simulink model "Demo919"  (R2018b)
settings: Solver=ode3  StartTime=0.0  StopTime=10  FixedStep=0.0005  RelTol=1e-3  EnableMultiTasking=on
values from neighbouring files (symbols this model uses):
  ADS1 = [1000 4000]    [data_new1.m]
  ADS2 = [900 4100]    [data_new1.m]
  br_opening = [0 20 40 60 80 100]    [data_new1.m]
  BRAKE = [485 1288 2091 2894 3697 4500]    [data_new1.m]
  InerWheel_Angle = [0 0.001 0.502 1.006 1.514 2.024 2.538 3.055 3.575 4.098 4.625 5.155 5.689 6.226 6.767 7.311 7.859 8.411 8.967 9.527 10.091 10.659 11.231 11.807 12.387 12.972 13.561 14.154 14.752 15.354 15.961 16.572 17.187 17.807 18.432 19.062 19.696 20.334 20.977 21.625 22.277 22.934 23.596 24.262 24.932 25.607 26.286 26.970 27.657 28.349 29.045 29.745 30.448 31.155 31.866]    [data_new1.m]
  OuterWheel_Angle = [0 0.001 0.501 1.001 1.501 2.001 2.501	3.001 3.501	4.001 4.501	5.001 5.501	6.001 6.501	7.001 7.501	8.001 8.501	9.001 9.501	10.001 10.501 11.001 11.501 12.001 12.501 13.001 13.501	14.001 14.501 15.001 15.501 16.001 16.501 17.001 17.501 18.001 18.501 19.001 19.501	20.001 20.501 21.001 21.501	22.001 22.501 23.001 23.501	24.001 24.501 25.001 25.501 26.001 26.501]    [data_new1.m]
  PUMP = [0 1000 2000 3000 4000 5000]    [data_new1.m]
  SteeringAngle_Cal = [-90 0 90]    [data_new1.m]
  SteeringAngle_Sensor = [640 1840 3041]    [data_new1.m]
  th_opening = [0 100]    [data_new1.m]
undefined symbols (not defined in the file or in its folder): D, I_AN06_5V, I_AN08_5V, I_AN09_5V, I_AN10_5V, I_HALL1, I_HALL2, I_SW01_L, I_SW10_L, I_SW11_H, I_SW12_H, I_SW13_H, I_SW14_H, I_SW15_H, I_SW16_H, I_SW17_H, I_SW18_H, I_SW19_H, I_SW20_H, O_PWM1_LS0A7, O_PWM2_LS0A7, O_SW02_LS0A4, O_SW13_HS1A, O_SW14_HS1A
libraries: ec5744lib x137, simulink x20, canmsglib x11
(part 4 of 5)

== system Demo919/Function-Call Subsystem1/Torque_Control/kongzhimokuai/FZ ==
  In1 : Inport
  In2 : Inport  Port=2
  Add3 : Sum
  Add4 : Sum
  Add7 : Sum
  Add8 : Sum  Inputs=+-
  Constant : Constant  Value=930
  Constant2 : Constant  Value=930
  Gain1 : Gain
  Gain11 : Gain
  Gain5 : Gain  Gain=33.17
  Gain6 : Gain  Gain=190.19
  Gain8 : Gain  Gain=33.17
  Gain9 : Gain  Gain=190.19
  k : Gain  Gain=14
  k1 : Gain  Gain=14
  Out1 : Outport
  Out2 : Outport  Port=2
  wires:
  Constant/1 -> Add7/2
  Add7/1 -> Add8/1
  k/1 -> Gain5/1
  Gain5/1 -> Add7/1
  Gain6/1 -> Add8/2
  Gain11/1 -> Gain6/1
  Add8/1 -> Out1/1
  In1/1 -> k1/1, k/1
  Gain1/1 -> Gain9/1
  Gain9/1 -> Add4/2
  Gain8/1 -> Add3/1
  k1/1 -> Gain8/1
  In2/1 -> Gain1/1, Gain11/1
  Add3/1 -> Add4/1
  Constant2/1 -> Add3/2
  Add4/1 -> Out2/1

== system Demo919/Function-Call Subsystem1/Torque_Control/kongzhimokuai/Filter1 ==
  note: 均值滤波器
  In1 : Inport
  Add2 : Sum  Inputs=-+-
  Gain2 : Gain  Gain=1/4
  MinMax : MinMax
  MinMax1 : MinMax  Function=max
  Sum of Elements : Sum  Inputs=+
  Tapped Delay : simulink/Discrete/Tapped Delay  vinit=0  samptime=-1  NumDelays=4  DelayOrder=Oldest  includeCurrent=off
  Out1 : Outport
  wires:
  Tapped Delay/1 -> Sum of Elements/1, MinMax1/1, MinMax/1
  Sum of Elements/1 -> Add2/2
  Gain2/1 -> Out1/1
  MinMax1/1 -> Add2/1
  MinMax/1 -> Add2/3
  Add2/1 -> Gain2/1
  In1/1 -> Tapped Delay/1

== system Demo919/Function-Call Subsystem1/Torque_Control/kongzhimokuai/Filter2 ==
  note: 均值滤波器
  In1 : Inport
  Add2 : Sum  Inputs=-+-
  Gain2 : Gain  Gain=1/4
  MinMax : MinMax
  MinMax1 : MinMax  Function=max
  Sum of Elements : Sum  Inputs=+
  Tapped Delay : simulink/Discrete/Tapped Delay  vinit=0.0  samptime=-1  NumDelays=6  DelayOrder=Oldest  includeCurrent=off
  Out1 : Outport
  wires:
  In1/1 -> Tapped Delay/1
  Add2/1 -> Gain2/1
  MinMax/1 -> Add2/3
  MinMax1/1 -> Add2/1
  Gain2/1 -> Out1/1
  Sum of Elements/1 -> Add2/2
  Tapped Delay/1 -> MinMax/1, MinMax1/1, Sum of Elements/1

== system Demo919/Function-Call Subsystem1/Torque_Control/kongzhimokuai/Filter3 ==
  note: 均值滤波器
  In1 : Inport
  Add2 : Sum  Inputs=-+-
  Gain2 : Gain  Gain=1/4
  MinMax : MinMax
  MinMax1 : MinMax  Function=max
  Sum of Elements : Sum  Inputs=+
  Tapped Delay : simulink/Discrete/Tapped Delay  vinit=0.0  samptime=-1  NumDelays=6  DelayOrder=Oldest  includeCurrent=off
  Out1 : Outport
  wires:
  Tapped Delay/1 -> Sum of Elements/1, MinMax1/1, MinMax/1
  Sum of Elements/1 -> Add2/2
  Gain2/1 -> Out1/1
  MinMax1/1 -> Add2/1
  MinMax/1 -> Add2/3
  Add2/1 -> Gain2/1
  In1/1 -> Tapped Delay/1

== system Demo919/Function-Call Subsystem1/Torque_Control/kongzhimokuai/Filter4 ==
  note: 均值滤波器
  In1 : Inport
  Add2 : Sum  Inputs=-+-
  Gain2 : Gain  Gain=1/4  OutDataTypeStr=double
  MinMax : MinMax
  MinMax1 : MinMax  Function=max
  Sum of Elements : Sum  Inputs=+
  Tapped Delay : simulink/Discrete/Tapped Delay  vinit=0  samptime=-1  NumDelays=4  DelayOrder=Oldest  includeCurrent=off
  Out1 : Outport
  wires:
  In1/1 -> Tapped Delay/1
  Add2/1 -> Gain2/1
  MinMax/1 -> Add2/3
  MinMax1/1 -> Add2/1
  Gain2/1 -> Out1/1
  Sum of Elements/1 -> Add2/2
  Tapped Delay/1 -> MinMax/1, MinMax1/1, Sum of Elements/1

== system Demo919/Function-Call Subsystem1/Torque_Control/kongzhimokuai/Filter5 ==
  note: 均值滤波器
  In1 : Inport
  Add2 : Sum  Inputs=-+-
  MinMax : MinMax
  MinMax1 : MinMax  Function=max
  Sum of Elements : Sum  Inputs=+
  Tapped Delay : simulink/Discrete/Tapped Delay  vinit=0  samptime=-1  NumDelays=3  DelayOrder=Oldest  includeCurrent=off
  Out1 : Outport
  wires:
  Tapped Delay/1 -> Sum of Elements/1, MinMax1/1, MinMax/1
  Sum of Elements/1 -> Add2/2
  Add2/1 -> Out1/1
  MinMax1/1 -> Add2/1
  MinMax/1 -> Add2/3
  In1/1 -> Tapped Delay/1

== system Demo919/Function-Call Subsystem1/Torque_Control/kongzhimokuai/Filter6 ==
  note: 均值滤波器
  In1 : Inport
  Add2 : Sum  Inputs=-+-
  MinMax : MinMax
  MinMax1 : MinMax  Function=max
  Sum of Elements : Sum  Inputs=+
  Tapped Delay : simulink/Discrete/Tapped Delay  vinit=0  samptime=-1  NumDelays=3  DelayOrder=Oldest  includeCurrent=off
  Out1 : Outport
  wires:
  Tapped Delay/1 -> Sum of Elements/1, MinMax1/1, MinMax/1
  Sum of Elements/1 -> Add2/2
  Add2/1 -> Out1/1
  MinMax1/1 -> Add2/1
  MinMax/1 -> Add2/3
  In1/1 -> Tapped Delay/1

== system Demo919/Function-Call Subsystem1/Torque_Control/kongzhimokuai/Fx ==
  In1 : Inport
  In2 : Inport  Port=2
  Add7 : Sum  Inputs=-+
  Add8 : Sum  Inputs=+-
  From96 : From  Commented=on  GotoTag=RolA21
  From97 : From  Commented=on  GotoTag=RolA22
  Gain5 : Gain  Gain=3.9
  Gain6 : Gain  Gain=3.9
  Jw : Constant  Commented=on  Value=0.235
  Jw1 : Constant  Commented=on  Value=0.235
  Product10 : Product  Commented=on
  Product11 : Product  Commented=on
  Out1 : Outport
  Out2 : Outport  Port=2
  wires:
  From96/1 -> Product10/2
  Gain5/1 -> Add8/1
  Product11/1 -> Add8/2
  Gain6/1 -> Add7/2
  Jw/1 -> Product10/1
  Jw1/1 -> Product11/2
  Product10/1 -> Add7/1
  From97/1 -> Product11/1
  In2/1 -> Gain5/1
  In1/1 -> Gain6/1
  Add7/1 -> Out1/1
  Add8/1 -> Out2/1

== system Demo919/Function-Call Subsystem1/Torque_Control/kongzhimokuai/Kalman_Filer ==
  In1 : Inport
  Data Type Conversion : DataTypeConversion  OutDataTypeStr=single
  Data Type Conversion1 : DataTypeConversion  OutDataTypeStr=single
  Delay : Delay  DelayLength=1  InitialCondition=0
  Delay1 : Delay  DelayLength=1  InitialCondition=0
  MATLAB Function : MATLAB Function  TreatAsAtomicUnit=on
  Out1 : Outport
  wires:
  In1/1 -> Data Type Conversion/1
  Data Type Conversion1/1 -> MATLAB Function/2(prevData)
  Data Type Conversion/1 -> MATLAB Function/1(inData)
  Delay/1 -> Data Type Conversion1/1
  MATLAB Function/1(inData_Output) -> Out1/1, Delay/1
  Delay1/1 -> MATLAB Function/3(Error)
  MATLAB Function/2(Error_Last) -> Delay1/1

== system Demo919/Function-Call Subsystem1/Torque_Control/kongzhimokuai/Kalman_Filer1 ==
  In1 : Inport
  Data Type Conversion : DataTypeConversion  OutDataTypeStr=single
  Data Type Conversion1 : DataTypeConversion  OutDataTypeStr=single
  Delay : Delay  DelayLength=1  InitialCondition=0
  Delay1 : Delay  DelayLength=1  InitialCondition=0
  MATLAB Function : MATLAB Function  TreatAsAtomicUnit=on
  Out1 : Outport
  wires:
  MATLAB Function/2(Error_Last) -> Delay1/1
  Delay1/1 -> MATLAB Function/3(Error)
  MATLAB Function/1(inData_Output) -> Delay/1, Out1/1
  Delay/1 -> Data Type Conversion1/1
  Data Type Conversion/1 -> MATLAB Function/1(inData)
  Data Type Conversion1/1 -> MATLAB Function/2(prevData)
  In1/1 -> Data Type Conversion/1

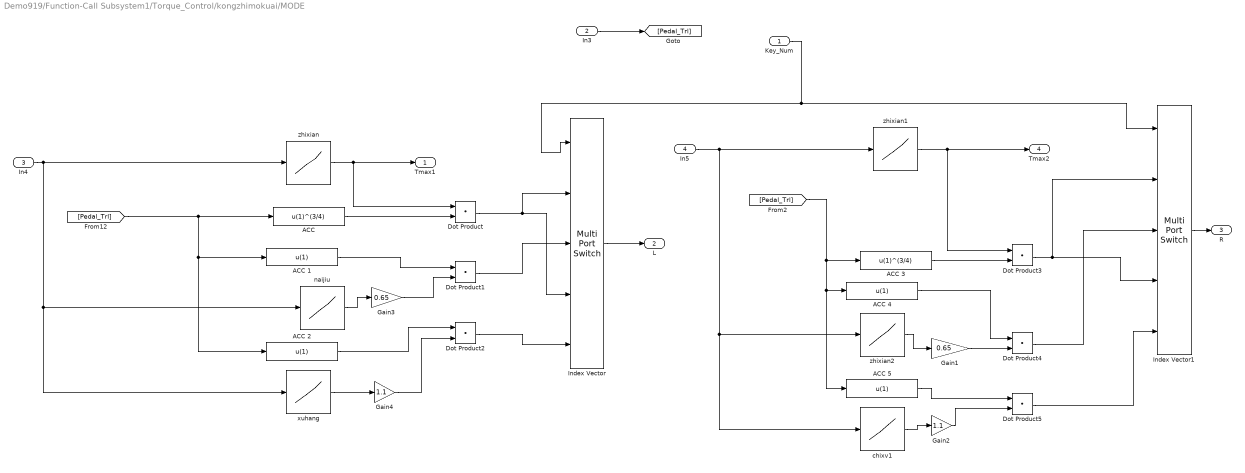
== system Demo919/Function-Call Subsystem1/Torque_Control/kongzhimokuai/MODE ==
  Key_Num : Inport
  In3 : Inport  Port=2
  In4 : Inport  Port=3
  In5 : Inport  Port=4
  "ACC " : Fcn  Expr=u(1)^(3/4)
  ACC {1..2,4..5} (4 alike) : Fcn  Expr=u(1)
  ACC 3 : Fcn  Expr=u(1)^(3/4)
  Dot Product{,1..5} (6 alike) : DotProduct  InputSameDT=on  OutDataTypeStr=Inherit: Inherit via internal rule
  Gain1 : Gain  Gain=0.65
  Gain2 : Gain  Gain=1.1
  Gain3 : Gain  Gain=0.65
  Gain4 : Gain  Gain=1.1
  Index Vector : MultiPortSwitch  DataPortOrder=Zero-based contiguous  Inputs=4  DiagnosticForDefault=None  zeroidx=on
  Index Vector1 : MultiPortSwitch  DataPortOrder=Zero-based contiguous  Inputs=4  DiagnosticForDefault=None  zeroidx=on
  chixv1 : Lookup_n-D  NumberOfTableDimensions=1  BreakpointsForDimension1=|  Table=|  InternalRulePriority=Speed  RndMeth=Simplest  InputSameDT=on
      BreakpointsForDimension1=|
      | [0
      | 44.6408100000000
      | 91.0709300000000
      | 138.722890000000
      | 182.709320000000
      | 229.139430000000
      | 274.347700000000
      | 321.999660000000
      | 364.764240000000
      | 411.194360000000
      | 460.068160000000
      | 504.054590000000
      | 550.484700000000
      | 596.914820000000
      | 640.901240000000
      | 687.331360000000
      | 732.539630000000
      | 780.191590000000
      | 822.956170000000
      | 871.829970000000
      | 918.260090000000
      | 964.690200000000
      | 1009.89847000000
      | 1053.88490000000
      | 1101.53686000000
      | 1149.18882000000
      | 1195.61894000000
      | 1239.60536000000
      | 1286.03548000000
      | 1333.68744000000
      | 1380.11755000000
      | 1425.32582000000
      | 1471.75594000000
      | 1516.96421000000
      | 1560.95063000000
      | 1608.60259000000
      | 1655.03271000000
      | 1701.46282000000
      | 1745.44925000000
      | 1791.87936000000
      | 1839.53132000000
      | 1885.96144000000
      | 1933.61340000000
      | 1977.59982000000
      | 2025.25178000000
      | 2071.68190000000
      | 2114.44648000000
      | 2163.32029000000
      | 2207.30671000000
      | 2253.73683000000
      | 2302.61063000000
      | 2346.59706000000
      | 2394.24902000000
      | 2439.45729000000
      | 2485.88740000000
      | 2531.09567000000
      | 2581.19132000000
      | 2626.39959000000
      | 2671.60786000000
      | 2718.03798000000
      | 2763.24625000000
      | 2809.67636000000
      | 2853.66279000000
      | 2898.87106000000
      | 2946.52302000000
      | 2994.17498000000
      | 3039.38325000000
      | 3085.81337000000
      | 3132.24348000000
      | 3178.67360000000
      | 3223.88187000000
      | 3270.31198000000
      | 3317.96394000000
      | 3363.17221000000
      | 3408.38048000000
      | 3453.58875000000
      | 3501.24071000000
      | 3546.44898000000
      | 3592.87910000000
      | 3639.30921000000
      | 3684.51748000000
      | 3729.72575000000
      | 3777.37771000000
      | 3822.58598000000
      | 3869.01610000000
      | 3915.44621000000
      | 3961.87633000000
      | 4008.30645000000
      | 4054.73656000000
      | 4101.16668000000
      | 4145.15310000000
      | 4192.80506000000
      | 4236.79149000000
      | 4285.66529000000
      | 4330.87356000000
      | 4374.85999000000
      | 4420.06826000000
      | 4466.49837000000
      | 4514.15033000000
      | 4559.35860000000
      | 4605.78872000000
      | 4650.99699000000
      | 4698.64895000000
      | 4743.85722000000
      | 4791.50918000000
      | 4834.27376000000
      | 4879.48203000000
      | 4925.91214000000
      | 4971.12041000000
      | 5019.99422000000
      | 5063.98065000000
      | 5112.85445000000
      | 5158.06272000000
      | 5202.04915000000
      | 5248.47926000000
      | 5294.90938000000
      | 5341.33949000000
      | 5388.99145000000
      | 5431.75603000000
      | 5478.18615000000
      | 5525.83811000000
      | 5569.82453000000
      | 5615.03280000000
      | 5662.68476000000
      | 5710.33672000000
      | 5753.10130000000
      | 5800.75326000000
      | 5848.40522000000
      | 5892.39165000000
      | 5938.82176000000
      | 6000]
      Table=|
      | [59.7747300000000
      | 59.9709300000000
      | 60.1671300000000
      | 60.4287400000000
      | 60.6249400000000
      | 60.8865500000000
      | 61.2135500000000
      | 61.4097600000000
      | 61.6059600000000
      | 61.8675700000000
      | 62.1945700000000
      | 62.3907800000000
      | 62.6523800000000
      | 62.9139900000000
      | 63.0447900000000
      | 63.2409900000000
      | 63.5680000000000
      | 63.7642000000000
      | 63.9604100000000
      | 64.2220100000000
      | 64.4182200000000
      | 64.6144200000000
      | 64.8106200000000
      | 64.9414300000000
      | 65.0068300000000
      | 65.2030300000000
      | 65.3338300000000
      | 65.4646400000000
      | 65.5300400000000
      | 65.6608400000000
      | 65.7916400000000
      | 65.9224400000000
      | 66.0532500000000
      | 66.1840500000000
      | 66.1840500000000
      | 66.2494500000000
      | 66.2494500000000
      | 66.2494500000000
      | 66.3802500000000
      | 66.4456500000000
      | 66.5764600000000
      | 66.7072600000000
      | 66.7072600000000
      | 66.7072600000000
      | 66.7072600000000
      | 66.7726600000000
      | 66.7726600000000
      | 66.8380600000000
      | 66.8380600000000
      | 66.9034600000000
      | 66.9688600000000
      | 66.9034600000000
      | 66.9034600000000
      | 66.9034600000000
      | 66.9688600000000
      | 67.0342700000000
      | 66.9688600000000
      | 66.9034600000000
      | 66.8380600000000
      | 66.7726600000000
      | 66.7072600000000
      | 66.7072600000000
      | 66.7072600000000
      | 66.7072600000000
      | 66.7072600000000
      | 66.6418600000000
      | 66.6418600000000
      | 66.6418600000000
      | 66.5764600000000
      | 66.5110600000000
      | 66.3802500000000
      | 66.2494500000000
      | 66.1840500000000
      | 66.1840500000000
      | 66.0532500000000
      | 66.0532500000000
      | 65.9878500000000
      | 65.8570400000000
      | 65.7262400000000
      | 65.6608400000000
      | 65.5954400000000
      | 65.4646400000000
      | 65.3992300000000
      | 65.2030300000000
      | 65.0722300000000
      | 64.9414300000000
      | 64.8106200000000
      | 64.6144200000000
      | 64.4836200000000
      | 64.3528100000000
      | 64.1566100000000
      | 63.8950100000000
      | 63.6334000000000
      | 63.5026000000000
      | 63.3063900000000
      | 63.0447900000000
      | 62.7831800000000
      | 62.4561800000000
      | 62.2599700000000
      | 62.0637700000000
      | 61.8021600000000
      | 61.6713600000000
      | 61.3443600000000
      | 61.1481500000000
      | 60.8211500000000
      | 60.5595400000000
      | 60.3633400000000
      | 60.1017300000000
      | 59.9055300000000
      | 59.5785200000000
      | 59.3823200000000
      | 59.1861100000000
      | 58.9899100000000
      | 58.7283100000000
      | 58.4667000000000
      | 58.2705000000000
      | 57.9434900000000
      | 57.6818900000000
      | 57.4856800000000
      | 57.3548800000000
      | 57.0932700000000
      | 56.8970700000000
      | 56.5046600000000
      | 56.2430600000000
      | 56.0468500000000
      | 55.9160500000000
      | 55.7852500000000
      | 55.5236400000000
      | 55.1966400000000
      | 54.9350300000000
      | 54.8042300000000]
  naijiu : Lookup_n-D  NumberOfTableDimensions=1  BreakpointsForDimension1=[0,45.86266,89.84908,137.50104,183.93116,230.36128,276.79139,321.99966,368.42978,413.63805,458.84632,506.49828,552.92839,598.13666,644.56678,690.99689,736.20516,785.07897,830.28724,876.71735,921.92562,969.57758,1014.78585,1061.21597,1106.42424,1154.0762,1198.06263,1244.49274,1292.1447,1337.35297,1383.78309,1431.43505,1476.64332,1521.85159,1570.72539,1613.48997,1662.36378,1705.12836,1752.78032,1800.43228,1846.86239,1892.07066,1937.27893,1983.70905,2028.91732,2075.34744,2122.9994,2166.98582,2214.63778,2261.0679,2306.27617,2353.92813,2397.91455,2444.34467,2490.77478,2535.98305,2583.63501,2630.06513,2676.49524,2721.70351,2766.91178,2814.56374,2858.55017,2906.20213,2951.4104,2999.06236,3045.49248,3090.70075,3137.13086,3183.56098,3228.76925,3275.19936,3322.85132,3366.83775,3412.04602,3459.69798,3506.12809,3553.78005,3600.21017,3641.7529,3690.62671,3735.83498,3782.26509,3828.69521,3873.90348,3920.3336,3965.54187,4011.97198,4058.4021,4104.83221,4151.26233,4197.69244,4242.90071,4290.55267,4332.09541,4379.74737,4427.39933,4471.38575,4519.03771,4561.80229,4609.45425,4655.88437,4701.09264,4747.52275,4791.50918,4836.71745,4881.92572,4928.35583,4973.56411,5019.99422,5065.20249,5110.41076,5155.61903,5198.38361,5244.81373,5290.022,5335.23027,5380.43854,5424.42496,5468.41139,5513.61966,5557.60608,5602.81435,5646.80078,5693.23089,5735.99547,5782.42559,5826.41201,5871.62028,5918.0504,6000]  Table=|  InternalRulePriority=Speed  RndMeth=Simplest  InputSameDT=on
      | [140
      | 139.695060000000
      | 139.695060000000
      | 139.629660000000
      | 139.564260000000
      | 139.498860000000
      | 139.433460000000
      | 139.368060000000
      | 139.302660000000
      | 139.237260000000
      | 139.171850000000
      | 139.171850000000
      | 139.171850000000
      | 139.106450000000
      | 139.041050000000
      | 139.041050000000
      | 138.975650000000
      | 138.975650000000
      | 138.779450000000
      | 138.779450000000
      | 138.714050000000
      | 138.648640000000
      | 138.517840000000
      | 138.452440000000
      | 138.517840000000
      | 138.517840000000
      | 138.452440000000
      | 138.452440000000
      | 138.387040000000
      | 138.321640000000
      | 138.321640000000
      | 138.256240000000
      | 138.190840000000
      | 138.060030000000
      | 138.060030000000
      | 138.060030000000
      | 137.994630000000
      | 137.929230000000
      | 137.929230000000
      | 137.863830000000
      | 137.798430000000
      | 137.733030000000
      | 137.667630000000
      | 137.667630000000
      | 137.667630000000
      | 137.602220000000
      | 137.602220000000
      | 137.536820000000
      | 137.471420000000
      | 137.536820000000
      | 137.340620000000
      | 137.340620000000
      | 137.275220000000
      | 137.275220000000
      | 137.209820000000
      | 137.144420000000
      | 137.144420000000
      | 137.079010000000
      | 136.948210000000
      | 136.882810000000
      | 136.882810000000
      | 136.948210000000
      | 136.752010000000
      | 136.817410000000
      | 136.752010000000
      | 136.686610000000
      | 136.555800000000
      | 136.555800000000
      | 136.490400000000
      | 136.490400000000
      | 136.425000000000
      | 136.359600000000
      | 136.294200000000
      | 136.163400000000
      | 136.097990000000
      | 136.032590000000
      | 136.032590000000
      | 135.901790000000
      | 135.836390000000
      | 135.770990000000
      | 135.705590000000
      | 135.574780000000
      | 135.443980000000
      | 135.313180000000
      | 135.116980000000
      | 134.986170000000
      | 134.789970000000
      | 134.593770000000
      | 134.397560000000
      | 134.201360000000
      | 133.939750000000
      | 133.678150000000
      | 133.481940000000
      | 133.220340000000
      | 132.958730000000
      | 132.631730000000
      | 132.435520000000
      | 132.108520000000
      | 131.716110000000
      | 131.389100000000
      | 131.062100000000
      | 130.735090000000
      | 130.277280000000
      | 130.015680000000
      | 129.623270000000
      | 129.230860000000
      | 128.773050000000
      | 128.380650000000
      | 127.922840000000
      | 127.530430000000
      | 127.007220000000
      | 126.484010000000
      | 125.960800000000
      | 125.437590000000
      | 124.979780000000
      | 124.391170000000
      | 123.802560000000
      | 123.213950000000
      | 122.625340000000
      | 122.036720000000
      | 121.317310000000
      | 120.728700000000
      | 120.074690000000
      | 119.616880000000
      | 118.832060000000
      | 118.374250000000
      | 117.654840000000
      | 117.131630000000
      | 116.477620000000
      | 115.823600000000
      | 115.234990000000]
  xuhang : Lookup_n-D  NumberOfTableDimensions=1  BreakpointsForDimension1=|  Table=|  InternalRulePriority=Speed  RndMeth=Simplest  InputSameDT=on
      BreakpointsForDimension1=|
      | [0
      | 44.6408100000000
      | 91.0709300000000
      | 138.722890000000
      | 182.709320000000
      | 229.139430000000
      | 274.347700000000
      | 321.999660000000
      | 364.764240000000
      | 411.194360000000
      | 460.068160000000
      | 504.054590000000
      | 550.484700000000
      | 596.914820000000
      | 640.901240000000
      | 687.331360000000
      | 732.539630000000
      | 780.191590000000
      | 822.956170000000
      | 871.829970000000
      | 918.260090000000
      | 964.690200000000
      | 1009.89847000000
      | 1053.88490000000
      | 1101.53686000000
      | 1149.18882000000
      | 1195.61894000000
      | 1239.60536000000
      | 1286.03548000000
      | 1333.68744000000
      | 1380.11755000000
      | 1425.32582000000
      | 1471.75594000000
      | 1516.96421000000
      | 1560.95063000000
      | 1608.60259000000
      | 1655.03271000000
      | 1701.46282000000
      | 1745.44925000000
      | 1791.87936000000
      | 1839.53132000000
      | 1885.96144000000
      | 1933.61340000000
      | 1977.59982000000
      | 2025.25178000000
      | 2071.68190000000
      | 2114.44648000000
      | 2163.32029000000
      | 2207.30671000000
      | 2253.73683000000
      | 2302.61063000000
      | 2346.59706000000
      | 2394.24902000000
      | 2439.45729000000
      | 2485.88740000000
      | 2531.09567000000
      | 2581.19132000000
      | 2626.39959000000
      | 2671.60786000000
      | 2718.03798000000
      | 2763.24625000000
      | 2809.67636000000
      | 2853.66279000000
      | 2898.87106000000
      | 2946.52302000000
      | 2994.17498000000
      | 3039.38325000000
      | 3085.81337000000
      | 3132.24348000000
      | 3178.67360000000
      | 3223.88187000000
      | 3270.31198000000
      | 3317.96394000000
      | 3363.17221000000
      | 3408.38048000000
      | 3453.58875000000
      | 3501.24071000000
      | 3546.44898000000
      | 3592.87910000000
      | 3639.30921000000
      | 3684.51748000000
      | 3729.72575000000
      | 3777.37771000000
      | 3822.58598000000
      | 3869.01610000000
      | 3915.44621000000
      | 3961.87633000000
      | 4008.30645000000
      | 4054.73656000000
      | 4101.16668000000
      | 4145.15310000000
      | 4192.80506000000
      | 4236.79149000000
      | 4285.66529000000
      | 4330.87356000000
      | 4374.85999000000
      | 4420.06826000000
      | 4466.49837000000
      | 4514.15033000000
      | 4559.35860000000
      | 4605.78872000000
      | 4650.99699000000
      | 4698.64895000000
      | 4743.85722000000
      | 4791.50918000000
      | 4834.27376000000
      | 4879.48203000000
      | 4925.91214000000
      | 4971.12041000000
      | 5019.99422000000
      | 5063.98065000000
      | 5112.85445000000
      | 5158.06272000000
      | 5202.04915000000
      | 5248.47926000000
      | 5294.90938000000
      | 5341.33949000000
      | 5388.99145000000
      | 5431.75603000000
      | 5478.18615000000
      | 5525.83811000000
      | 5569.82453000000
      | 5615.03280000000
      | 5662.68476000000
      | 5710.33672000000
      | 5753.10130000000
      | 5800.75326000000
      | 5848.40522000000
      | 5892.39165000000
      | 5938.82176000000
      | 6000]
      Table=|
      | [59.7747300000000
      | 59.9709300000000
      | 60.1671300000000
      | 60.4287400000000
      | 60.6249400000000
      | 60.8865500000000
      | 61.2135500000000
      | 61.4097600000000
      | 61.6059600000000
      | 61.8675700000000
      | 62.1945700000000
      | 62.3907800000000
      | 62.6523800000000
      | 62.9139900000000
      | 63.0447900000000
      | 63.2409900000000
      | 63.5680000000000
      | 63.7642000000000
      | 63.9604100000000
      | 64.2220100000000
      | 64.4182200000000
      | 64.6144200000000
      | 64.8106200000000
      | 64.9414300000000
      | 65.0068300000000
      | 65.2030300000000
      | 65.3338300000000
      | 65.4646400000000
      | 65.5300400000000
      | 65.6608400000000
      | 65.7916400000000
      | 65.9224400000000
      | 66.0532500000000
      | 66.1840500000000
      | 66.1840500000000
      | 66.2494500000000
      | 66.2494500000000
      | 66.2494500000000
      | 66.3802500000000
      | 66.4456500000000
      | 66.5764600000000
      | 66.7072600000000
      | 66.7072600000000
      | 66.7072600000000
      | 66.7072600000000
      | 66.7726600000000
      | 66.7726600000000
      | 66.8380600000000
      | 66.8380600000000
      | 66.9034600000000
      | 66.9688600000000
      | 66.9034600000000
      | 66.9034600000000
      | 66.9034600000000
      | 66.9688600000000
      | 67.0342700000000
      | 66.9688600000000
      | 66.9034600000000
      | 66.8380600000000
      | 66.7726600000000
      | 66.7072600000000
      | 66.7072600000000
      | 66.7072600000000
      | 66.7072600000000
      | 66.7072600000000
      | 66.6418600000000
      | 66.6418600000000
      | 66.6418600000000
      | 66.5764600000000
      | 66.5110600000000
      | 66.3802500000000
      | 66.2494500000000
      | 66.1840500000000
      | 66.1840500000000
      | 66.0532500000000
      | 66.0532500000000
      | 65.9878500000000
      | 65.8570400000000
      | 65.7262400000000
      | 65.6608400000000
      | 65.5954400000000
      | 65.4646400000000
      | 65.3992300000000
      | 65.2030300000000
      | 65.0722300000000
      | 64.9414300000000
      | 64.8106200000000
      | 64.6144200000000
      | 64.4836200000000
      | 64.3528100000000
      | 64.1566100000000
      | 63.8950100000000
      | 63.6334000000000
      | 63.5026000000000
      | 63.3063900000000
      | 63.0447900000000
      | 62.7831800000000
      | 62.4561800000000
      | 62.2599700000000
      | 62.0637700000000
      | 61.8021600000000
      | 61.6713600000000
      | 61.3443600000000
      | 61.1481500000000
      | 60.8211500000000
      | 60.5595400000000
      | 60.3633400000000
      | 60.1017300000000
      | 59.9055300000000
      | 59.5785200000000
      | 59.3823200000000
      | 59.1861100000000
      | 58.9899100000000
      | 58.7283100000000
      | 58.4667000000000
      | 58.2705000000000
      | 57.9434900000000
      | 57.6818900000000
      | 57.4856800000000
      | 57.3548800000000
      | 57.0932700000000
      | 56.8970700000000
      | 56.5046600000000
      | 56.2430600000000
      | 56.0468500000000
      | 55.9160500000000
      | 55.7852500000000
      | 55.5236400000000
      | 55.1966400000000
      | 54.9350300000000
      | 54.8042300000000]
  zhixian : Lookup_n-D  NumberOfTableDimensions=1  BreakpointsForDimension1=[0,45.86266,89.84908,137.50104,183.93116,230.36128,276.79139,321.99966,368.42978,413.63805,458.84632,506.49828,552.92839,598.13666,644.56678,690.99689,736.20516,785.07897,830.28724,876.71735,921.92562,969.57758,1014.78585,1061.21597,1106.42424,1154.0762,1198.06263,1244.49274,1292.1447,1337.35297,1383.78309,1431.43505,1476.64332,1521.85159,1570.72539,1613.48997,1662.36378,1705.12836,1752.78032,1800.43228,1846.86239,1892.07066,1937.27893,1983.70905,2028.91732,2075.34744,2122.9994,2166.98582,2214.63778,2261.0679,2306.27617,2353.92813,2397.91455,2444.34467,2490.77478,2535.98305,2583.63501,2630.06513,2676.49524,2721.70351,2766.91178,2814.56374,2858.55017,2906.20213,2951.4104,2999.06236,3045.49248,3090.70075,3137.13086,3183.56098,3228.76925,3275.19936,3322.85132,3366.83775,3412.04602,3459.69798,3506.12809,3553.78005,3600.21017,3641.7529,3690.62671,3735.83498,3782.26509,3828.69521,3873.90348,3920.3336,3965.54187,4011.97198,4058.4021,4104.83221,4151.26233,4197.69244,4242.90071,4290.55267,4332.09541,4379.74737,4427.39933,4471.38575,4519.03771,4561.80229,4609.45425,4655.88437,4701.09264,4747.52275,4791.50918,4836.71745,4881.92572,4928.35583,4973.56411,5019.99422,5065.20249,5110.41076,5155.61903,5198.38361,5244.81373,5290.022,5335.23027,5380.43854,5424.42496,5468.41139,5513.61966,5557.60608,5602.81435,5646.80078,5693.23089,5735.99547,5782.42559,5826.41201,5871.62028,5918.0504,6000]  Table=|  InternalRulePriority=Speed  RndMeth=Simplest  InputSameDT=on
      | [140
      | 139.695060000000
      | 139.695060000000
      | 139.629660000000
      | 139.564260000000
      | 139.498860000000
      | 139.433460000000
      | 139.368060000000
      | 139.302660000000
      | 139.237260000000
      | 139.171850000000
      | 139.171850000000
      | 139.171850000000
      | 139.106450000000
      | 139.041050000000
      | 139.041050000000
      | 138.975650000000
      | 138.975650000000
      | 138.779450000000
      | 138.779450000000
      | 138.714050000000
      | 138.648640000000
      | 138.517840000000
      | 138.452440000000
      | 138.517840000000
      | 138.517840000000
      | 138.452440000000
      | 138.452440000000
      | 138.387040000000
      | 138.321640000000
      | 138.321640000000
      | 138.256240000000
      | 138.190840000000
      | 138.060030000000
      | 138.060030000000
      | 138.060030000000
      | 137.994630000000
      | 137.929230000000
      | 137.929230000000
      | 137.863830000000
      | 137.798430000000
      | 137.733030000000
      | 137.667630000000
      | 137.667630000000
      | 137.667630000000
      | 137.602220000000
      | 137.602220000000
      | 137.536820000000
      | 137.471420000000
      | 137.536820000000
      | 137.340620000000
      | 137.340620000000
      | 137.275220000000
      | 137.275220000000
      | 137.209820000000
      | 137.144420000000
      | 137.144420000000
      | 137.079010000000
      | 136.948210000000
      | 136.882810000000
      | 136.882810000000
      | 136.948210000000
      | 136.752010000000
      | 136.817410000000
      | 136.752010000000
      | 136.686610000000
      | 136.555800000000
      | 136.555800000000
      | 136.490400000000
      | 136.490400000000
      | 136.425000000000
      | 136.359600000000
      | 136.294200000000
      | 136.163400000000
      | 136.097990000000
      | 136.032590000000
      | 136.032590000000
      | 135.901790000000
      | 135.836390000000
      | 135.770990000000
      | 135.705590000000
      | 135.574780000000
      | 135.443980000000
      | 135.313180000000
      | 135.116980000000
      | 134.986170000000
      | 134.789970000000
      | 134.593770000000
      | 134.397560000000
      | 134.201360000000
      | 133.939750000000
      | 133.678150000000
      | 133.481940000000
      | 133.220340000000
      | 132.958730000000
      | 132.631730000000
      | 132.435520000000
      | 132.108520000000
      | 131.716110000000
      | 131.389100000000
      | 131.062100000000
      | 130.735090000000
      | 130.277280000000
      | 130.015680000000
      | 129.623270000000
      | 129.230860000000
      | 128.773050000000
      | 128.380650000000
      | 127.922840000000
      | 127.530430000000
      | 127.007220000000
      | 126.484010000000
      | 125.960800000000
      | 125.437590000000
      | 124.979780000000
      | 124.391170000000
      | 123.802560000000
      | 123.213950000000
      | 122.625340000000
      | 122.036720000000
      | 121.317310000000
      | 120.728700000000
      | 120.074690000000
      | 119.616880000000
      | 118.832060000000
      | 118.374250000000
      | 117.654840000000
      | 117.131630000000
      | 116.477620000000
      | 115.823600000000
      | 115.234990000000]
  zhixian1 : Lookup_n-D  NumberOfTableDimensions=1  BreakpointsForDimension1=[0,45.86266,89.84908,137.50104,183.93116,230.36128,276.79139,321.99966,368.42978,413.63805,458.84632,506.49828,552.92839,598.13666,644.56678,690.99689,736.20516,785.07897,830.28724,876.71735,921.92562,969.57758,1014.78585,1061.21597,1106.42424,1154.0762,1198.06263,1244.49274,1292.1447,1337.35297,1383.78309,1431.43505,1476.64332,1521.85159,1570.72539,1613.48997,1662.36378,1705.12836,1752.78032,1800.43228,1846.86239,1892.07066,1937.27893,1983.70905,2028.91732,2075.34744,2122.9994,2166.98582,2214.63778,2261.0679,2306.27617,2353.92813,2397.91455,2444.34467,2490.77478,2535.98305,2583.63501,2630.06513,2676.49524,2721.70351,2766.91178,2814.56374,2858.55017,2906.20213,2951.4104,2999.06236,3045.49248,3090.70075,3137.13086,3183.56098,3228.76925,3275.19936,3322.85132,3366.83775,3412.04602,3459.69798,3506.12809,3553.78005,3600.21017,3641.7529,3690.62671,3735.83498,3782.26509,3828.69521,3873.90348,3920.3336,3965.54187,4011.97198,4058.4021,4104.83221,4151.26233,4197.69244,4242.90071,4290.55267,4332.09541,4379.74737,4427.39933,4471.38575,4519.03771,4561.80229,4609.45425,4655.88437,4701.09264,4747.52275,4791.50918,4836.71745,4881.92572,4928.35583,4973.56411,5019.99422,5065.20249,5110.41076,5155.61903,5198.38361,5244.81373,5290.022,5335.23027,5380.43854,5424.42496,5468.41139,5513.61966,5557.60608,5602.81435,5646.80078,5693.23089,5735.99547,5782.42559,5826.41201,5871.62028,5918.0504,6000]  Table=|  InternalRulePriority=Speed  RndMeth=Simplest  InputSameDT=on
      | [140
      | 139.695060000000
      | 139.695060000000
      | 139.629660000000
      | 139.564260000000
      | 139.498860000000
      | 139.433460000000
      | 139.368060000000
      | 139.302660000000
      | 139.237260000000
      | 139.171850000000
      | 139.171850000000
      | 139.171850000000
      | 139.106450000000
      | 139.041050000000
      | 139.041050000000
      | 138.975650000000
      | 138.975650000000
      | 138.779450000000
      | 138.779450000000
      | 138.714050000000
      | 138.648640000000
      | 138.517840000000
      | 138.452440000000
      | 138.517840000000
      | 138.517840000000
      | 138.452440000000
      | 138.452440000000
      | 138.387040000000
      | 138.321640000000
      | 138.321640000000
      | 138.256240000000
      | 138.190840000000
      | 138.060030000000
      | 138.060030000000
      | 138.060030000000
      | 137.994630000000
      | 137.929230000000
      | 137.929230000000
      | 137.863830000000
      | 137.798430000000
      | 137.733030000000
      | 137.667630000000
      | 137.667630000000
      | 137.667630000000
      | 137.602220000000
      | 137.602220000000
      | 137.536820000000
      | 137.471420000000
      | 137.536820000000
      | 137.340620000000
      | 137.340620000000
      | 137.275220000000
      | 137.275220000000
      | 137.209820000000
      | 137.144420000000
      | 137.144420000000
      | 137.079010000000
      | 136.948210000000
      | 136.882810000000
      | 136.882810000000
      | 136.948210000000
      | 136.752010000000
      | 136.817410000000
      | 136.752010000000
      | 136.686610000000
      | 136.555800000000
      | 136.555800000000
      | 136.490400000000
      | 136.490400000000
      | 136.425000000000
      | 136.359600000000
      | 136.294200000000
      | 136.163400000000
      | 136.097990000000
      | 136.032590000000
      | 136.032590000000
      | 135.901790000000
      | 135.836390000000
      | 135.770990000000
      | 135.705590000000
      | 135.574780000000
      | 135.443980000000
      | 135.313180000000
      | 135.116980000000
      | 134.986170000000
      | 134.789970000000
      | 134.593770000000
      | 134.397560000000
      | 134.201360000000
      | 133.939750000000
      | 133.678150000000
      | 133.481940000000
      | 133.220340000000
      | 132.958730000000
      | 132.631730000000
      | 132.435520000000
      | 132.108520000000
      | 131.716110000000
      | 131.389100000000
      | 131.062100000000
      | 130.735090000000
      | 130.277280000000
      | 130.015680000000
      | 129.623270000000
      | 129.230860000000
      | 128.773050000000
      | 128.380650000000
      | 127.922840000000
      | 127.530430000000
      | 127.007220000000
      | 126.484010000000
      | 125.960800000000
      | 125.437590000000
      | 124.979780000000
      | 124.391170000000
      | 123.802560000000
      | 123.213950000000
      | 122.625340000000
      | 122.036720000000
      | 121.317310000000
      | 120.728700000000
      | 120.074690000000
      | 119.616880000000
      | 118.832060000000
      | 118.374250000000
      | 117.654840000000
      | 117.131630000000
      | 116.477620000000
      | 115.823600000000
      | 115.234990000000]
  zhixian2 : Lookup_n-D  NumberOfTableDimensions=1  BreakpointsForDimension1=[0,45.86266,89.84908,137.50104,183.93116,230.36128,276.79139,321.99966,368.42978,413.63805,458.84632,506.49828,552.92839,598.13666,644.56678,690.99689,736.20516,785.07897,830.28724,876.71735,921.92562,969.57758,1014.78585,1061.21597,1106.42424,1154.0762,1198.06263,1244.49274,1292.1447,1337.35297,1383.78309,1431.43505,1476.64332,1521.85159,1570.72539,1613.48997,1662.36378,1705.12836,1752.78032,1800.43228,1846.86239,1892.07066,1937.27893,1983.70905,2028.91732,2075.34744,2122.9994,2166.98582,2214.63778,2261.0679,2306.27617,2353.92813,2397.91455,2444.34467,2490.77478,2535.98305,2583.63501,2630.06513,2676.49524,2721.70351,2766.91178,2814.56374,2858.55017,2906.20213,2951.4104,2999.06236,3045.49248,3090.70075,3137.13086,3183.56098,3228.76925,3275.19936,3322.85132,3366.83775,3412.04602,3459.69798,3506.12809,3553.78005,3600.21017,3641.7529,3690.62671,3735.83498,3782.26509,3828.69521,3873.90348,3920.3336,3965.54187,4011.97198,4058.4021,4104.83221,4151.26233,4197.69244,4242.90071,4290.55267,4332.09541,4379.74737,4427.39933,4471.38575,4519.03771,4561.80229,4609.45425,4655.88437,4701.09264,4747.52275,4791.50918,4836.71745,4881.92572,4928.35583,4973.56411,5019.99422,5065.20249,5110.41076,5155.61903,5198.38361,5244.81373,5290.022,5335.23027,5380.43854,5424.42496,5468.41139,5513.61966,5557.60608,5602.81435,5646.80078,5693.23089,5735.99547,5782.42559,5826.41201,5871.62028,5918.0504,6000]  Table=|  InternalRulePriority=Speed  RndMeth=Simplest  InputSameDT=on
      | [140
      | 139.695060000000
      | 139.695060000000
      | 139.629660000000
      | 139.564260000000
      | 139.498860000000
      | 139.433460000000
      | 139.368060000000
      | 139.302660000000
      | 139.237260000000
      | 139.171850000000
      | 139.171850000000
      | 139.171850000000
      | 139.106450000000
      | 139.041050000000
      | 139.041050000000
      | 138.975650000000
      | 138.975650000000
      | 138.779450000000
      | 138.779450000000
      | 138.714050000000
      | 138.648640000000
      | 138.517840000000
      | 138.452440000000
      | 138.517840000000
      | 138.517840000000
      | 138.452440000000
      | 138.452440000000
      | 138.387040000000
      | 138.321640000000
      | 138.321640000000
      | 138.256240000000
      | 138.190840000000
      | 138.060030000000
      | 138.060030000000
      | 138.060030000000
      | 137.994630000000
      | 137.929230000000
      | 137.929230000000
      | 137.863830000000
      | 137.798430000000
      | 137.733030000000
      | 137.667630000000
      | 137.667630000000
      | 137.667630000000
      | 137.602220000000
      | 137.602220000000
      | 137.536820000000
      | 137.471420000000
      | 137.536820000000
      | 137.340620000000
      | 137.340620000000
      | 137.275220000000
      | 137.275220000000
      | 137.209820000000
      | 137.144420000000
      | 137.144420000000
      | 137.079010000000
      | 136.948210000000
      | 136.882810000000
      | 136.882810000000
      | 136.948210000000
      | 136.752010000000
      | 136.817410000000
      | 136.752010000000
      | 136.686610000000
      | 136.555800000000
      | 136.555800000000
      | 136.490400000000
      | 136.490400000000
      | 136.425000000000
      | 136.359600000000
      | 136.294200000000
      | 136.163400000000
      | 136.097990000000
      | 136.032590000000
      | 136.032590000000
      | 135.901790000000
      | 135.836390000000
      | 135.770990000000
      | 135.705590000000
      | 135.574780000000
      | 135.443980000000
      | 135.313180000000
      | 135.116980000000
      | 134.986170000000
      | 134.789970000000
      | 134.593770000000
      | 134.397560000000
      | 134.201360000000
      | 133.939750000000
      | 133.678150000000
      | 133.481940000000
      | 133.220340000000
      | 132.958730000000
      | 132.631730000000
      | 132.435520000000
      | 132.108520000000
      | 131.716110000000
      | 131.389100000000
      | 131.062100000000
      | 130.735090000000
      | 130.277280000000
      | 130.015680000000
      | 129.623270000000
      | 129.230860000000
      | 128.773050000000
      | 128.380650000000
      | 127.922840000000
      | 127.530430000000
      | 127.007220000000
      | 126.484010000000
      | 125.960800000000
      | 125.437590000000
      | 124.979780000000
      | 124.391170000000
      | 123.802560000000
      | 123.213950000000
      | 122.625340000000
      | 122.036720000000
      | 121.317310000000
      | 120.728700000000
      | 120.074690000000
      | 119.616880000000
      | 118.832060000000
      | 118.374250000000
      | 117.654840000000
      | 117.131630000000
      | 116.477620000000
      | 115.823600000000
      | 115.234990000000]
  Tmax1 : Outport
  L : Outport  Port=2
  R : Outport  Port=3
  Tmax2 : Outport  Port=4
  wires:
  In4/1 -> zhixian/1, xuhang/1, naijiu/1
  [Pedal_Trl] -> ACC 2/1, ACC 1/1, "ACC "/1
  ACC 1/1 -> Dot Product1/1
  xuhang/1 -> Gain4/1
  Key_Num/1 -> Index Vector/1, Index Vector1/1
  Dot Product1/1 -> Index Vector/3
  ACC 2/1 -> Dot Product2/1
  "ACC "/1 -> Dot Product/2
  naijiu/1 -> Gain3/1
  Gain4/1 -> Dot Product2/2
  Gain3/1 -> Dot Product1/2
  In3/1 -> [Pedal_Trl]
  Index Vector/1 -> L/1
  Gain1/1 -> Dot Product4/2
  Gain2/1 -> Dot Product5/2
  zhixian2/1 -> Gain1/1
  ACC 3/1 -> Dot Product3/2
  ACC 5/1 -> Dot Product5/1
  chixv1/1 -> Gain2/1
  ACC 4/1 -> Dot Product4/1
  In5/1 -> zhixian1/1, zhixian2/1, chixv1/1
  zhixian/1 -> Tmax1/1, Dot Product/1
  zhixian1/1 -> Tmax2/1, Dot Product3/1
  Dot Product/1 -> Index Vector/2, Index Vector/4
  Dot Product3/1 -> Index Vector1/2, Index Vector1/4
  [Pedal_Trl] -> ACC 3/1, ACC 4/1, ACC 5/1
  Dot Product2/1 -> Index Vector/5
  Dot Product5/1 -> Index Vector1/5
  Dot Product4/1 -> Index Vector1/3
  Index Vector1/1 -> R/1

== system Demo919/Function-Call Subsystem1/Torque_Control/kongzhimokuai/OQ_2 ==
  In1 : Inport
  Bitwise Operator : simulink/Logic and Bit Operations/Bitwise Operator  logicop=AND  UseBitMask=on  BitMask=bin2dec('11111111')  BitMaskRealWorld=Stored Integer
  Data Type Conversion : DataTypeConversion  OutDataTypeStr=uint8
  Data Type Conversion1 : DataTypeConversion  OutDataTypeStr=uint8
  Shift Arithmetic : ArithShift  BitShiftNumber=8  BitShiftDirection=Right
  Mot_TorqH : Outport
  Mot_TorqL : Outport  Port=2
  wires:
  Data Type Conversion1/1 -> Mot_TorqL/1
  Bitwise Operator/1 -> Data Type Conversion1/1
  Data Type Conversion/1 -> Mot_TorqH/1
  Shift Arithmetic/1 -> Data Type Conversion/1
  In1/1 -> Shift Arithmetic/1, Bitwise Operator/1

== system Demo919/Function-Call Subsystem1/Torque_Control/kongzhimokuai/OQ_3 ==
  In1 : Inport
  Bitwise Operator : simulink/Logic and Bit Operations/Bitwise Operator  logicop=AND  UseBitMask=on  BitMask=bin2dec('11111111')  BitMaskRealWorld=Stored Integer
  Data Type Conversion : DataTypeConversion  OutDataTypeStr=uint8
  Data Type Conversion1 : DataTypeConversion  OutDataTypeStr=uint8
  Shift Arithmetic : ArithShift  BitShiftNumber=8  BitShiftDirection=Right
  Mot_TorqH : Outport
  Mot_TorqL : Outport  Port=2
  wires:
  In1/1 -> Bitwise Operator/1, Shift Arithmetic/1
  Shift Arithmetic/1 -> Data Type Conversion/1
  Data Type Conversion/1 -> Mot_TorqH/1
  Bitwise Operator/1 -> Data Type Conversion1/1
  Data Type Conversion1/1 -> Mot_TorqL/1

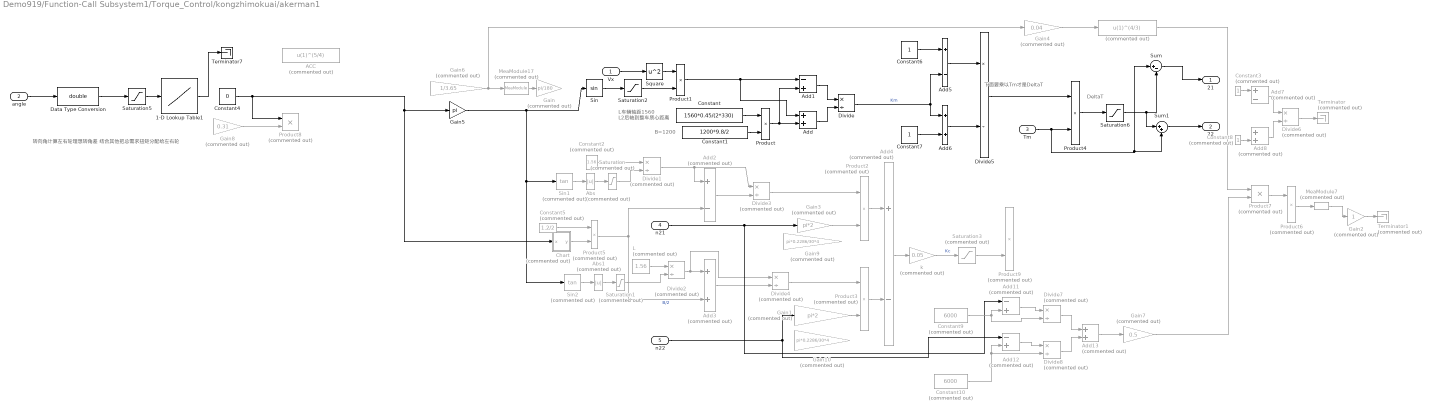
== system Demo919/Function-Call Subsystem1/Torque_Control/kongzhimokuai/akerman1 ==
  note: B=1200
  note: DeltaT
  note: 下面要乘以Tm才是DeltaT
  note: L车辆轴距1560
      | L2后轴到整车质心距离
  note: 转向角计算左右轮理想转角差
      | 结合其他把总需求扭矩分配给左右轮
  "Vx " : Inport
  angle : Inport  Port=2
  "Tm " : Inport  Port=3
  n21 : Inport  Port=4
  n22 : Inport  Port=5
  " " : Fcn  Commented=on  Expr=u(1)^(4/3)
  1-D Lookup Table1 : Lookup_n-D  NumberOfTableDimensions=1  BreakpointsForDimension1=[50 1175 2300]  Table=[1 0 -1]  InternalRulePriority=Speed  RndMeth=Simplest  InputSameDT=on
  "ACC " : Fcn  Commented=on  Expr=u(1)^(5/4)
  Abs : Abs  Commented=on
  Abs1 : Abs  Commented=on
  Add : Sum
  Add1 : Sum  Inputs=-+
  Add11 : Sum  Commented=on  Inputs=-+
  Add12 : Sum  Commented=on  Inputs=-+
  Add13 : Sum  Commented=on
  Add2 : Sum  Commented=on  Inputs=+-
  Add3 : Sum  Commented=on
  Add4 : Sum  Commented=on  Inputs=+-
  Add5 : Sum  Inputs=+-
  Add6 : Sum
  Add7 : Sum  Commented=on  Inputs=+-
  Add8 : Sum  Commented=on
  Chart : Stateflow chart  Commented=on  TreatAsAtomicUnit=on
  Constant : Constant  Value=1560*0.45/(2*330)
  Constant1 : Constant  Value=1200*9.8/2
  Constant10 : Constant  Commented=on  Value=6000
  Constant2 : Constant  Commented=on  Value=1.56
  Constant3 : Constant  Commented=on
  Constant4 : Constant  Value=0
  Constant5 : Constant  Commented=on  Value=1.2/2
  Constant6 : Constant
  Constant7 : Constant
  Constant8 : Constant  Commented=on
  Constant9 : Constant  Commented=on  Value=6000
  Data Type Conversion : DataTypeConversion  OutDataTypeStr=double
  Divide : Product  Inputs=*/
  Divide{1..4,6..8} (7 alike) : Product  Commented=on  Inputs=*/
  Divide5 : Product  Inputs=*/
  Gain : Gain  Commented=on  Gain=pi/180
  Gain1 : Gain  Commented=on  Gain=pi*2
  Gain10 : Gain  Commented=on  Gain=pi*0.2286/30*4
  Gain2 : Gain  Commented=on
  Gain3 : Gain  Commented=on  Gain=pi*2
  Gain4 : Gain  Commented=on  Gain=0.04
  Gain5 : Gain  Gain=pi
  Gain6 : Gain  Commented=on  Gain=1/3.65  OutDataTypeStr=double
  Gain7 : Gain  Commented=on  Gain=0.5
  Gain8 : Gain  Commented=on  Gain=0.31
  Gain9 : Gain  Commented=on  Gain=pi*0.2286/30*4
  L : Constant  Commented=on  Value=1.56
  MeaModule17 : ec5744lib/RapidECU_U3/07Calibration/MeaModule  Commented=on  signal=b8
      settings: SourceProductName=ECUCoder for MPC5744
  MeaModule7 : ec5744lib/RapidECU_U3/07Calibration/MeaModule  Commented=on  signal=d6
      settings: SourceProductName=ECUCoder for MPC5744
  Product : Product
  Product1 : Product
  Product{2..3,5..9} (7 alike) : Product  Commented=on
  Product4 : Product
  Saturation : Saturate  Commented=on  UpperLimit=2.59  LowerLimit=0.173
  Saturation1 : Saturate  Commented=on  UpperLimit=2.59  LowerLimit=0.173
  Saturation2 : Saturate  UpperLimit=1  LowerLimit=-1
  Saturation3 : Saturate  Commented=on  UpperLimit=1  LowerLimit=-1
  Saturation5 : Saturate  UpperLimit=2300  LowerLimit=50
  Saturation6 : Saturate  UpperLimit=2  LowerLimit=-2
  Sin : Trigonometry
  Sin1 : Trigonometry  Commented=on  Operator=tan
  Sin2 : Trigonometry  Commented=on  Operator=tan
  Square : Math  Operator=square  SaturateOnIntegerOverflow=on
  Sum : Sum  Inputs=|+-
  Sum1 : Sum  Inputs=|++
  Terminator : Terminator  Commented=on
  Terminator1 : Terminator  Commented=on
  Terminator7 : Terminator
  k : Gain  Commented=on  Gain=0.05
  21 : Outport
  "22 " : Outport  Port=2
  wires:
  Divide6/1 -> Terminator/1
  Gain3/1 -> Product2/2
  Product7/1 -> Product6/1
  Gain4/1 -> " "/1
  " "/1 -> Product7/1
  Divide5/1 -> Product4/1
  Sin/1 -> Saturation2/1
  Constant/1 -> Product/1
  Constant1/1 -> Product/2
  "Vx "/1 -> Square/1
  Square/1 -> Product1/1
  Product1/1 -> Add/1, Add1/1
  Product/1 -> Add/2, Add1/2
  Add1/1 -> Divide/1
  Add/1 -> Divide/2
  Constant2/1 -> Divide1/1
  Divide1/1 -> Divide3/1, Add2/1
  Product5/1 -> Add3/2, Add2/2  "B/2"
  L/1 -> Divide2/1
  Add2/1 -> Divide3/2
  Divide2/1 -> Add3/1, Divide4/1
  Add3/1 -> Divide4/2
  Product2/1 -> Add4/1
  Product3/1 -> Add4/2
  Divide/1 -> Add5/2, Add6/1  "Km"
  Constant6/1 -> Add5/1
  Constant7/1 -> Add6/2
  Add5/1 -> Divide5/1
  Add6/1 -> Divide5/2
  Add4/1 -> k/1
  Gain1/1 -> Product3/2
  Chart/1(y) -> Product5/2
  Constant5/1 -> Product5/1
  k/1 -> Saturation3/1  "Kc"
  Abs/1 -> Saturation/1
  Sin1/1 -> Abs/1
  Saturation/1 -> Divide1/2
  Abs1/1 -> Saturation1/1
  Sin2/1 -> Abs1/1
  Saturation1/1 -> Divide2/2
  Constant3/1 -> Add7/1
  Constant8/1 -> Add8/2
  Add7/1 -> Divide6/1
  Add8/1 -> Divide6/2
  Divide3/1 -> Product2/1
  Divide4/1 -> Product3/1
  Saturation2/1 -> Product1/2
  Product6/1 -> MeaModule7/1
  Gain6/1 -> MeaModule17/1, Gain4/1
  angle/1 -> Data Type Conversion/1
  MeaModule17/1 -> Gain/1
  Data Type Conversion/1 -> Saturation5/1
  Saturation5/1 -> 1-D Lookup Table1/1
  MeaModule7/1 -> Gain2/1
  n21/1 -> Add11/1, Gain3/1
  Divide8/1 -> Add13/2
  Constant10/1 -> Add12/2, Divide8/2
  Add12/1 -> Divide8/1
  Constant9/1 -> Divide7/2, Add11/2
  n22/1 -> Gain1/1, Add12/1
  Divide7/1 -> Add13/1
  Add11/1 -> Divide7/1
  Add13/1 -> Gain7/1
  Gain7/1 -> Product7/2
  Constant4/1 -> Gain5/1, Chart/1(x), Product8/1
  Gain8/1 -> Product8/2
  Gain2/1 -> Terminator1/1
  Gain5/1 -> Sin/1, Sin2/1, Sin1/1
  "Tm "/1 -> Sum1/2, Sum/1, Product4/2
  Saturation3/1 -> Product9/2
  Sum/1 -> 21/1
  Sum1/1 -> "22 "/1
  Product4/1 -> Saturation6/1
  Saturation6/1 -> Sum1/1, Sum/2
  1-D Lookup Table1/1 -> Terminator7/1
